simulink model "aaa"  (R2016b)
settings: Solver=ode4  StartTime=0.0  StopTime=inf  FixedStep=0.002  RelTol=1e-3  EnableMultiTasking=on
undefined symbols (not defined in the file or in its folder): bit, mdaadlink6208, sigbuilder_block, Standard
libraries: slrtlib x20, slrtsoftinglib x11, simulink x10
(part 3 of 4)

== system aaa/Subsystem2/zidong/Subsystem ==
  kaigaikaishi : Inport
  guangaikaishi : Inport  Port=2
  kaigaiquxian : Inport  Port=3
  guangaiquxian : Inport  Port=4
  xkgg : Inport  Port=5
  Add1 : Sum
  Constant : Constant  Value=2
  Constant1 : Constant  Value=-0.05
  Display{,1..3} (4 alike) : Display
  Gain : Gain  Gain=0.15
  Gain1 : Gain  Gain=0.15
  Multiport Switch : MultiPortSwitch
  Product : Product
  Sum : Sum  Inputs=|+-
  Sum1 : Sum  Inputs=|+-
  Out1 : Outport
  wires:
  guangaikaishi/1 -> Product/1
  Constant/1 -> Product/2
  kaigaikaishi/1 -> Add1/1
  Product/1 -> Add1/2
  Add1/1 -> Multiport Switch/1
  Multiport Switch/1 -> Display2/1, Out1/1
  Sum/1 -> Gain/1
  Gain/1 -> Multiport Switch/2, Display1/1
  Sum1/1 -> Gain1/1
  Gain1/1 -> Display/1, Multiport Switch/3
  Constant1/1 -> Multiport Switch/4
  xkgg/1 -> Display3/1, Sum1/2, Sum/2
  kaigaiquxian/1 -> Sum/1
  guangaiquxian/1 -> Sum1/1

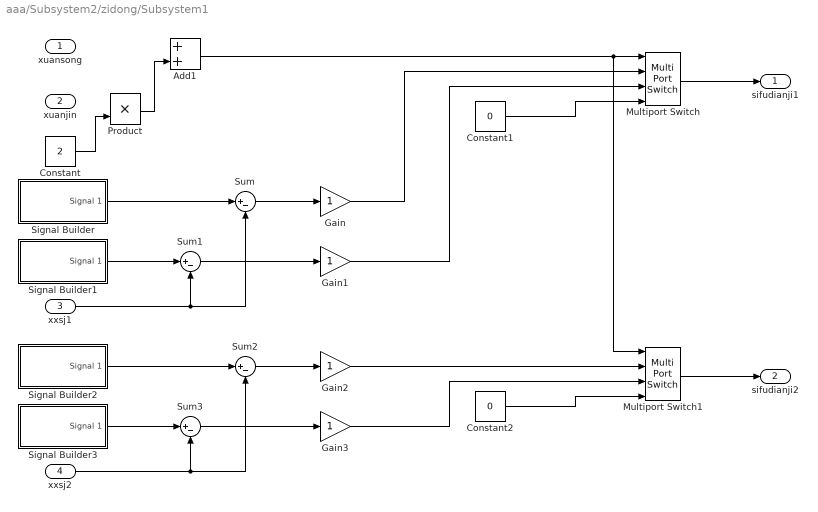
== system aaa/Subsystem2/zidong/Subsystem1 ==
  xuansong : Inport
  xuanjin : Inport  Port=2
  xxsj1 : Inport  Port=3
  xxsj2 : Inport  Port=4
  Add1 : Sum
  Constant : Constant  Value=2
  Constant1 : Constant  Value=0
  Constant2 : Constant  Value=0
  Gain{,1..3} (4 alike) : Gain
  Multiport Switch : MultiPortSwitch
  Multiport Switch1 : MultiPortSwitch
  Product : Product
  Signal Builder : Subsystem  Tag=STV Subsys  LoadFcn=sigbuilder_block('load');  StartFcn=sigbuilder_block('start');  StopFcn=sigbuilder_block('stop');  ClipboardFcn=sigbuilder_block('clipboard');  mask(Sigbuilder block){tuvar=[0:10]}
      mask help: Simulink:masks:SigbuilderBlock_MD
      mask init:
      | if ~strcmp(get_param(bdroot(gcbh),'SimulationStatus'),'stopped') tuvar = sigbuilder_block('maskInit'); end
      settings: CopyFcn=sigbuilder_block('copy');  DeleteFcn=sigbuilder_block('delete');  ModelCloseFcn=sigbuilder_block('modelClose');  PreSaveFcn=sigbuilder_block('preSave');  PauseFcn=sigbuilder_block('pause');  ContinueFcn=sigbuilder_block('continue');  NameChangeFcn=sigbuilder_block('namechange');  OpenFcn=sigbuilder_block('open',[437.6 199.2 550.4 400 ]);  CloseFcn=sigbuilder_block('close');
      mask Display: plot(0, 0, 100, 100,[2, 2, 32, 32, 2], [68, 8, 8, 68, 68],[32, 2], [38, 38], [32, 19, 2],[53, 60, 44], [32, 17, 17, 2],[16, 16, 31, 31]);txt = getActiveGroup(gcbh);text(2, 100, txt,'verticalAlignment', 'top');
  Signal Builder1 : Subsystem  Tag=STV Subsys  LoadFcn=sigbuilder_block('load');  StartFcn=sigbuilder_block('start');  StopFcn=sigbuilder_block('stop');  ClipboardFcn=sigbuilder_block('clipboard');  mask(Sigbuilder block){tuvar=[0:10]}
      mask help: Simulink:masks:SigbuilderBlock_MD
      mask init:
      | if ~strcmp(get_param(bdroot(gcbh),'SimulationStatus'),'stopped') tuvar = sigbuilder_block('maskInit'); end
      settings: CopyFcn=sigbuilder_block('copy');  DeleteFcn=sigbuilder_block('delete');  ModelCloseFcn=sigbuilder_block('modelClose');  PreSaveFcn=sigbuilder_block('preSave');  PauseFcn=sigbuilder_block('pause');  ContinueFcn=sigbuilder_block('continue');  NameChangeFcn=sigbuilder_block('namechange');  OpenFcn=sigbuilder_block('open',[437.6 199.2 550.4 400 ]);  CloseFcn=sigbuilder_block('close');
      mask Display: plot(0, 0, 100, 100,[2, 2, 32, 32, 2], [68, 8, 8, 68, 68],[32, 2], [38, 38], [32, 19, 2],[53, 60, 44], [32, 17, 17, 2],[16, 16, 31, 31]);txt = getActiveGroup(gcbh);text(2, 100, txt,'verticalAlignment', 'top');
  Signal Builder2 : Subsystem  Tag=STV Subsys  LoadFcn=sigbuilder_block('load');  StartFcn=sigbuilder_block('start');  StopFcn=sigbuilder_block('stop');  ClipboardFcn=sigbuilder_block('clipboard');  mask(Sigbuilder block){tuvar=[0:10]}
      mask help: Simulink:masks:SigbuilderBlock_MD
      mask init:
      | if ~strcmp(get_param(bdroot(gcbh),'SimulationStatus'),'stopped') tuvar = sigbuilder_block('maskInit'); end
      settings: CopyFcn=sigbuilder_block('copy');  DeleteFcn=sigbuilder_block('delete');  ModelCloseFcn=sigbuilder_block('modelClose');  PreSaveFcn=sigbuilder_block('preSave');  PauseFcn=sigbuilder_block('pause');  ContinueFcn=sigbuilder_block('continue');  NameChangeFcn=sigbuilder_block('namechange');  OpenFcn=sigbuilder_block('open',[437.6 199.2 550.4 400 ]);  CloseFcn=sigbuilder_block('close');
      mask Display: plot(0, 0, 100, 100,[2, 2, 32, 32, 2], [68, 8, 8, 68, 68],[32, 2], [38, 38], [32, 19, 2],[53, 60, 44], [32, 17, 17, 2],[16, 16, 31, 31]);txt = getActiveGroup(gcbh);text(2, 100, txt,'verticalAlignment', 'top');
  Signal Builder3 : Subsystem  Tag=STV Subsys  LoadFcn=sigbuilder_block('load');  StartFcn=sigbuilder_block('start');  StopFcn=sigbuilder_block('stop');  ClipboardFcn=sigbuilder_block('clipboard');  mask(Sigbuilder block){tuvar=[0:10]}
      mask help: Simulink:masks:SigbuilderBlock_MD
      mask init:
      | if ~strcmp(get_param(bdroot(gcbh),'SimulationStatus'),'stopped') tuvar = sigbuilder_block('maskInit'); end
      settings: CopyFcn=sigbuilder_block('copy');  DeleteFcn=sigbuilder_block('delete');  ModelCloseFcn=sigbuilder_block('modelClose');  PreSaveFcn=sigbuilder_block('preSave');  PauseFcn=sigbuilder_block('pause');  ContinueFcn=sigbuilder_block('continue');  NameChangeFcn=sigbuilder_block('namechange');  OpenFcn=sigbuilder_block('open',[437.6 199.2 550.4 400 ]);  CloseFcn=sigbuilder_block('close');
      mask Display: plot(0, 0, 100, 100,[2, 2, 32, 32, 2], [68, 8, 8, 68, 68],[32, 2], [38, 38], [32, 19, 2],[53, 60, 44], [32, 17, 17, 2],[16, 16, 31, 31]);txt = getActiveGroup(gcbh);text(2, 100, txt,'verticalAlignment', 'top');
  Sum{,1..3} (4 alike) : Sum  Inputs=|+-
  sifudianji1 : Outport
  sifudianji2 : Outport  Port=2
  wires:
  Constant1/1 -> Multiport Switch/4
  Gain1/1 -> Multiport Switch/3
  Sum1/1 -> Gain1/1
  Signal Builder1/1(Signal 1) -> Sum1/1
  Gain/1 -> Multiport Switch/2
  Sum/1 -> Gain/1
  xxsj1/1 -> Sum/2, Sum1/2
  Signal Builder/1(Signal 1) -> Sum/1
  Multiport Switch/1 -> sifudianji1/1
  Add1/1 -> Multiport Switch1/1, Multiport Switch/1
  Product/1 -> Add1/2
  Constant/1 -> Product/2
  Multiport Switch1/1 -> sifudianji2/1
  Signal Builder2/1(Signal 1) -> Sum2/1
  xxsj2/1 -> Sum2/2, Sum3/2
  Sum2/1 -> Gain2/1
  Gain2/1 -> Multiport Switch1/2
  Signal Builder3/1(Signal 1) -> Sum3/1
  Sum3/1 -> Gain3/1
  Gain3/1 -> Multiport Switch1/3
  Constant2/1 -> Multiport Switch1/4

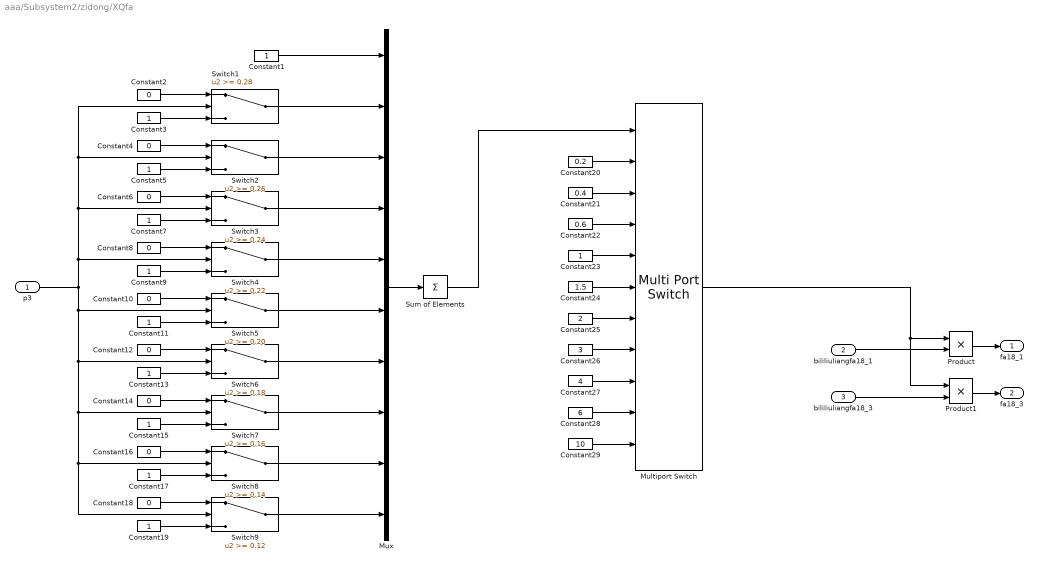
== system aaa/Subsystem2/zidong/XQfa ==
  p3 : Inport
  bililiuliangfa18_1 : Inport  Port=2
  bililiuliangfa18_3 : Inport  Port=3
  Constant{1,3,5,7,9,11,13,15,17,19,23} (11 alike) : Constant
  Constant{2,4,6,8,10,12,14,16,18} (9 alike) : Constant  Value=0
  Constant20 : Constant  Value=0.2
  Constant21 : Constant  Value=0.4
  Constant22 : Constant  Value=0.6
  Constant24 : Constant  Value=1.5
  Constant25 : Constant  Value=2
  Constant26 : Constant  Value=3
  Constant27 : Constant  Value=4
  Constant28 : Constant  Value=6
  Constant29 : Constant  Value=10
  Multiport Switch : MultiPortSwitch  Inputs=10
  Mux : Mux  Inputs=10
  Product : Product  RndMeth=Zero
  Product1 : Product  RndMeth=Zero
  Sum of Elements : Sum  Inputs=+
  Switch1 : Switch  Threshold=0.28
  Switch2 : Switch  Threshold=0.26
  Switch3 : Switch  Threshold=0.24
  Switch4 : Switch  Threshold=0.22
  Switch5 : Switch  Threshold=0.20
  Switch6 : Switch  Threshold=0.18
  Switch7 : Switch  Threshold=0.16
  Switch8 : Switch  Threshold=0.14
  Switch9 : Switch  Threshold=0.12
  fa18_1 : Outport
  fa18_3 : Outport  Port=2
  wires:
  Constant2/1 -> Switch1/1
  Constant3/1 -> Switch1/3
  Constant4/1 -> Switch2/1
  Constant5/1 -> Switch2/3
  Constant6/1 -> Switch3/1
  Constant7/1 -> Switch3/3
  Constant8/1 -> Switch4/1
  Constant9/1 -> Switch4/3
  Constant10/1 -> Switch5/1
  Constant11/1 -> Switch5/3
  Constant12/1 -> Switch6/1
  Constant13/1 -> Switch6/3
  Constant14/1 -> Switch7/1
  Constant15/1 -> Switch7/3
  p3/1 -> Switch1/2, Switch2/2, Switch3/2, Switch4/2, Switch6/2, Switch7/2, Switch8/2, Switch9/2, Switch5/2
  Mux/1 -> Sum of Elements/1
  Sum of Elements/1 -> Multiport Switch/1
  Constant1/1 -> Mux/1
  Switch1/1 -> Mux/2
  Switch2/1 -> Mux/3
  Switch3/1 -> Mux/4
  Switch4/1 -> Mux/5
  Switch5/1 -> Mux/6
  Switch6/1 -> Mux/7
  Switch7/1 -> Mux/8
  Switch8/1 -> Mux/9
  Switch9/1 -> Mux/10
  Constant16/1 -> Switch8/1
  Constant17/1 -> Switch8/3
  Constant18/1 -> Switch9/1
  Constant19/1 -> Switch9/3
  Multiport Switch/1 -> Product/1, Product1/1
  Constant20/1 -> Multiport Switch/2
  Constant21/1 -> Multiport Switch/3
  Constant22/1 -> Multiport Switch/4
  Constant23/1 -> Multiport Switch/5
  Constant24/1 -> Multiport Switch/6
  Constant25/1 -> Multiport Switch/7
  Constant26/1 -> Multiport Switch/8
  Constant27/1 -> Multiport Switch/9
  Constant28/1 -> Multiport Switch/10
  Constant29/1 -> Multiport Switch/11
  bililiuliangfa18_1/1 -> Product/2
  bililiuliangfa18_3/1 -> Product1/2
  Product/1 -> fa18_1/1
  Product1/1 -> fa18_3/1

== system aaa/Subsystem2/shoudong/Subsystem2/Signal Builder ==
  Demux : Demux  Tag=STV Demux  Outputs=1
  FromWs : FromWorkspace  Tag=STV FromWs  VariableName=tuvar  SampleTime=0
      SigBuilderData=|
      | common.afterFinalStr = 'Extrapolate'
      | common.sampleTime = 0
      | dataSet.timeRange = [0 10]
      | dataSet.name = 'Group 1'
      | sbobj.Groups.Name = 'Group 1'
      | sbobj.Groups.Signals.Name = 'Signal 1'
      | sbobj.Groups.Signals.XData = [0 4 4 6 6 10]
      | sbobj.Groups.Signals.YData = [0 0 1 1 0 0]
  Signal 1 : Outport  Tag=STV Outport
  wires:
  FromWs/1 -> Demux/1
  Demux/1 -> Signal 1/1

== system aaa/Subsystem2/shoudong/Subsystem2/Signal Builder1 ==
  Demux : Demux  Tag=STV Demux  Outputs=1
  FromWs : FromWorkspace  Tag=STV FromWs  VariableName=tuvar  SampleTime=0
      SigBuilderData=|
      | common.afterFinalStr = 'Extrapolate'
      | common.sampleTime = 0
      | dataSet.timeRange = [0 10]
      | dataSet.name = 'Group 1'
      | sbobj.Groups.Name = 'Group 1'
      | sbobj.Groups.Signals.Name = 'Signal 1'
      | sbobj.Groups.Signals.XData = [0 4 4 6 6 10]
      | sbobj.Groups.Signals.YData = [0 0 1 1 0 0]
  Signal 1 : Outport  Tag=STV Outport
  wires:
  Demux/1 -> Signal 1/1
  FromWs/1 -> Demux/1

== system aaa/Subsystem2/shoudong/Subsystem2/Signal Builder2 ==
  Demux : Demux  Tag=STV Demux  Outputs=1
  FromWs : FromWorkspace  Tag=STV FromWs  VariableName=tuvar  SampleTime=0
      SigBuilderData=|
      | common.afterFinalStr = 'Extrapolate'
      | common.sampleTime = 0
      | dataSet.timeRange = [0 10]
      | dataSet.name = 'Group 1'
      | sbobj.Groups.Name = 'Group 1'
      | sbobj.Groups.Signals.Name = 'Signal 1'
      | sbobj.Groups.Signals.XData = [0 4 4 6 6 10]
      | sbobj.Groups.Signals.YData = [0 0 1 1 0 0]
  Signal 1 : Outport  Tag=STV Outport
  wires:
  Demux/1 -> Signal 1/1
  FromWs/1 -> Demux/1

== system aaa/Subsystem2/shoudong/Subsystem2/Signal Builder3 ==
  Demux : Demux  Tag=STV Demux  Outputs=1
  FromWs : FromWorkspace  Tag=STV FromWs  VariableName=tuvar  SampleTime=0
      SigBuilderData=|
      | common.afterFinalStr = 'Extrapolate'
      | common.sampleTime = 0
      | dataSet.timeRange = [0 10]
      | dataSet.name = 'Group 1'
      | sbobj.Groups.Name = 'Group 1'
      | sbobj.Groups.Signals.Name = 'Signal 1'
      | sbobj.Groups.Signals.XData = [0 4 4 6 6 10]
      | sbobj.Groups.Signals.YData = [0 0 1 1 0 0]
  Signal 1 : Outport  Tag=STV Outport
  wires:
  FromWs/1 -> Demux/1
  Demux/1 -> Signal 1/1

== system aaa/Subsystem2/zidong/Subsystem1/Signal Builder ==
  Demux : Demux  Tag=STV Demux  Outputs=1
  FromWs : FromWorkspace  Tag=STV FromWs  VariableName=tuvar  SampleTime=0
      SigBuilderData=|
      | common.afterFinalStr = 'Extrapolate'
      | common.sampleTime = 0
      | dataSet.timeRange = [0 10]
      | dataSet.name = 'Group 1'
      | sbobj.Groups.Name = 'Group 1'
      | sbobj.Groups.Signals.Name = 'Signal 1'
      | sbobj.Groups.Signals.XData = [0 4 4 6 6 10]
      | sbobj.Groups.Signals.YData = [0 0 1 1 0 0]
  Signal 1 : Outport  Tag=STV Outport
  wires:
  FromWs/1 -> Demux/1
  Demux/1 -> Signal 1/1

== system aaa/Subsystem2/zidong/Subsystem1/Signal Builder1 ==
  Demux : Demux  Tag=STV Demux  Outputs=1
  FromWs : FromWorkspace  Tag=STV FromWs  VariableName=tuvar  SampleTime=0
      SigBuilderData=|
      | common.afterFinalStr = 'Extrapolate'
      | common.sampleTime = 0
      | dataSet.timeRange = [0 10]
      | dataSet.name = 'Group 1'
      | sbobj.Groups.Name = 'Group 1'
      | sbobj.Groups.Signals.Name = 'Signal 1'
      | sbobj.Groups.Signals.XData = [0 4 4 6 6 10]
      | sbobj.Groups.Signals.YData = [0 0 1 1 0 0]
  Signal 1 : Outport  Tag=STV Outport
  wires:
  Demux/1 -> Signal 1/1
  FromWs/1 -> Demux/1

== system aaa/Subsystem2/zidong/Subsystem1/Signal Builder2 ==
  Demux : Demux  Tag=STV Demux  Outputs=1
  FromWs : FromWorkspace  Tag=STV FromWs  VariableName=tuvar  SampleTime=0
      SigBuilderData=|
      | common.afterFinalStr = 'Extrapolate'
      | common.sampleTime = 0
      | dataSet.timeRange = [0 10]
      | dataSet.name = 'Group 1'
      | sbobj.Groups.Name = 'Group 1'
      | sbobj.Groups.Signals.Name = 'Signal 1'
      | sbobj.Groups.Signals.XData = [0 4 4 6 6 10]
      | sbobj.Groups.Signals.YData = [0 0 1 1 0 0]
  Signal 1 : Outport  Tag=STV Outport
  wires:
  Demux/1 -> Signal 1/1
  FromWs/1 -> Demux/1

== system aaa/Subsystem2/zidong/Subsystem1/Signal Builder3 ==
  Demux : Demux  Tag=STV Demux  Outputs=1
  FromWs : FromWorkspace  Tag=STV FromWs  VariableName=tuvar  SampleTime=0
      SigBuilderData=|
      | common.afterFinalStr = 'Extrapolate'
      | common.sampleTime = 0
      | dataSet.timeRange = [0 10]
      | dataSet.name = 'Group 1'
      | sbobj.Groups.Name = 'Group 1'
      | sbobj.Groups.Signals.Name = 'Signal 1'
      | sbobj.Groups.Signals.XData = [0 4 4 6 6 10]
      | sbobj.Groups.Signals.YData = [0 0 1 1 0 0]
  Signal 1 : Outport  Tag=STV Outport
  wires:
  FromWs/1 -> Demux/1
  Demux/1 -> Signal 1/1

== stateflow chart aaa/Subsystem2/zidong/Chart ==
  state zidong
    state SXQxieya
      state off1
        entry:
        diancifa11_1=0;
        bililiuliangfa18_3=0;
        bililiuliangfa18_4=0;
      state on1
        entry:
        diancifa11_5=1;
      state xieya1
        entry:
        bililiuliangfa18_1=1;
        bililiuliangfa18_2=1;
        p0_2=p0sheding;
      state xieya1_2
        entry:
        bililiuliangfa18_1=1;
        bililiuliangfa18_2=0;
      state xieya1_1
        entry:
        bililiuliangfa18_1=1;
        bililiuliangfa18_2=1;
      state xieya1_3
        entry:
        bililiuliangfa18_1=0;
        bililiuliangfa18_2=1;
      state xieya2
        entry:
        bililiuliangfa18_1=1;
        bililiuliangfa18_2=1;
        p0_2=p0_2-0.03;
      state xieya7_2
        entry:
        bililiuliangfa18_1=1;
        bililiuliangfa18_2=0;
      state xieya7_1
        entry:
        bililiuliangfa18_1=1;
        bililiuliangfa18_2=1;
      state xieya7_3
        entry:
        bililiuliangfa18_1=0;
        bililiuliangfa18_2=1;
      state off2
        entry:
        diancifa11_5=0;
        bililiuliangfa18_1=0;
        bililiuliangfa18_2=0;
        SXQxieyawancheng=1;
      state xieya8
        entry:
        bililiuliangfa18_1=1;
        bililiuliangfa18_2=1;
      (default) -> zidong.SXQxieya.off1
      zidong.SXQxieya.off1 -> zidong.SXQxieya.on1
      zidong.SXQxieya.on1 -> xieya1 : after(20,tick)
      xieya1 -> (junction 1107)
      (junction 1107) -> xieya1_2 [order 2] : [p2<=p0_2&&p3>p0_2]
      (junction 1107) -> xieya1_1 [order 1] : [p2>p0_2&&p3>p0_2]
      xieya1_2 -> (junction 1107)
      xieya1_3 -> (junction 1107)
      xieya1_1 -> (junction 1107)
      (junction 1107) -> xieya1_3 [order 3] : [p2>p0_2&&p3<=p0_2]
      (junction 1107) -> xieya2 [order 4] : [p2<=p0_2&&p3<=p0_2]
      (junction 1108) -> (junction 1107) [order 2] : [p0_2>p0_0]
      xieya2 -> (junction 1108)
      (junction 1108) -> (junction 1109) [order 1] : [p0_2<=p0_0]
      (junction 1109) -> xieya7_2 [order 2] : [p2<=p0_0&&p3>p0_0]
      xieya7_2 -> (junction 1109)
      (junction 1109) -> xieya7_1 [order 1] : [p2>p0_0&&p3>p0_0]
      xieya7_3 -> (junction 1109)
      (junction 1109) -> xieya7_3 [order 3] : [p2>p0_0&&p3<=p0_0]
      xieya7_1 -> (junction 1109)
      (junction 1109) -> xieya8 [order 4] : [p2<=p0_0&&p3<=p0_0]
      (junction 1110) -> (junction 1109) [order 2] : [p2>p0_0||p3>p0_0]
      (junction 1110) -> zidong.SXQxieya.off2 [order 1] : [p2<=p0_0&&p3<=p0_0]
      xieya8 -> (junction 1110) : after(1000,tick)
    state kaiguangai
      state start
        entry:
        xuansong=0;
        xuanjin=0;
        suoding=0;
        jiesuo=0;
        kaigaikaishi=0;
        guangaikaishi=0;
        diancifa20=0;
      state on5
        entry:
        jiesuo=1;
        xuansong=1;
      state off5
        entry:
        jiesuo=0;
        xuansong=0;
      state on1
        entry:diancifa20=1;
      state on6
        entry:
        guangaikaishi=1;
      state on2
        entry:
        xuansong=1;
        jiesuo=1;
      state on7
        entry:
        guangaikaishi=0;
        diancifa20=1;
      state off1
        entry:
        xuansong=0;
        jiesuo=0;
      state on8
        entry:
        xuanjin=1;
      state off2
        entry:
        diancifa20=0;
        SQshiyabuchangwancheng=1;
      state off6
        entry:
        xuanjin=0;
      state on3
        entry:
        kaigaikaishi=1;
      state on4
        entry:
        kaigaikaishi=0;
        suoding=1;
      state off7
        entry:
        diancifa20=0;
        SQxuanjinjianyawancheng=1;
        guangaiwancheng=1;
      state off3
        entry:
        suoding=0;
      state off4
        entry:
        kaigaiwancheng=1;
      (default) -> zidong.kaiguangai.start
      zidong.kaiguangai.off4 -> on5 : after(2500,tick)
      on5 -> off5 : [jiesuodaowei1==1&&jiesuodaowei2==1&&xuansongdaowei1==1&&xuansongdaowei2==1]
      zidong.kaiguangai.start -> zidong.kaiguangai.on1
      off5 -> on6 : after(500,tick)
      zidong.kaiguangai.on1 -> zidong.kaiguangai.on2 : [liuliangji==1&&p1>=p2-0.01&&p1<=p2+0.01]
      on6 -> on7 : [guangaijieshu==1]
      zidong.kaiguangai.on2 -> zidong.kaiguangai.off1 : [xuansongdaowei1==1&&xuansongdaowei2==1&&jiesuodaowei1==1&&jiesuodaowei2==1]
      on7 -> on8
      zidong.kaiguangai.off1 -> zidong.kaiguangai.off2 : after(20,tick)
      on8 -> zidong.kaiguangai.off6 : [xuanjindaowei1==1&&xuanjindaowei2==1]
      zidong.kaiguangai.off2 -> zidong.kaiguangai.on3 : after(500,tick)
      zidong.kaiguangai.off6 -> off7 : after(20,tick)
      zidong.kaiguangai.on3 -> on4 : [kaigaijieshu==1]
      on4 -> zidong.kaiguangai.off3 : [suodingdaowei1==1&&suodingdaowei2==1]
      zidong.kaiguangai.off3 -> zidong.kaiguangai.off4 : after(20,tick)
    state SCjiaya
      state off1
        entry:diancifa11_1=0;
        diancifa11_2=0;
        diancifa16_1=0;
      state on1
        entry:diancifa11_1=1;
        diancifa11_2=1;
        diancifa16_1=0;
      state off2
        entry:
        diancifa11_1=0;
        diancifa11_2=0;
        diancifa16_1=0;
      state on3
        entry:diancifa11_1=1;
        diancifa11_2=1;
        diancifa16_1=0;
      state on2
        entry:diancifa16_1=1;
      state off3
        entry:
        diancifa11_1=0;
        diancifa11_2=0;
        diancifa16_1=0;
      state off4
        entry:
        SCjiayawancheng=1;
      (default) -> zidong.SCjiaya.off1
      zidong.SCjiaya.off1 -> zidong.SCjiaya.on1
      zidong.SCjiaya.on1 -> zidong.SCjiaya.off2 : [p1>=p1sheding]
      zidong.SCjiaya.off2 -> (junction 45) : after(1000,tick)
      zidong.SCjiaya.on2 -> (junction 45)
      zidong.SCjiaya.on3 -> (junction 45)
      (junction 45) -> zidong.SCjiaya.on2 [order 2] : [p1>p1sheding+0.005]
      (junction 45) -> zidong.SCjiaya.on3 [order 1] : [p1<p1sheding]
      (junction 45) -> zidong.SCjiaya.off3 [order 3] : [p1>=p1sheding&&p1<=p1sheding+0.005]
      zidong.SCjiaya.off3 -> zidong.SCjiaya.off4
    state SCzhushui
      state off4
        entry:diancifa16_1=0;
        diancifa3=0;
      state on2
        entry:diancifa16_1=1;
      state on3
        entry:diancifa3=1;
      state off1
        entry:diancifa3=0;
      state off2
        entry:diancifa16_1=0;
      state off3
        entry:
        SCzhushuiwancheng=1;
      (default) -> zidong.SCzhushui.off4
      zidong.SCzhushui.off4 -> zidong.SCzhushui.on2
      zidong.SCzhushui.on2 -> zidong.SCzhushui.on3 : after(20,tick)
      zidong.SCzhushui.on3 -> zidong.SCzhushui.off1 : [fuqiuyeweikongzhiqi==1]
      zidong.SCzhushui.off1 -> zidong.SCzhushui.off2
      zidong.SCzhushui.off2 -> zidong.SCzhushui.off3
    state SXQjunya
      state jiaya1_1
        entry:
        bililiuliangfa18_3=1;
        bililiuliangfa18_4=1;
      state jiaya7_1
        entry:
        bililiuliangfa18_3=1;
        bililiuliangfa18_4=1;
      state jiaya7_3
        entry:
        bililiuliangfa18_3=0;
        bililiuliangfa18_4=1;
      state jiaya2
        entry:
        bililiuliangfa18_3=1;
        bililiuliangfa18_4=1;
        p0_1=p0_1+0.03;
      state off1
        entry:
        diancifa11_1=0;
        diancifa11_5=0;
        diancifa20=0;
        bililiuliangfa18_1=0;
        bililiuliangfa18_2=0;
        bililiuliangfa18_3=0;
        bililiuliangfa18_4=0;
      state jiaya1
        entry:
        bililiuliangfa18_3=1;
        bililiuliangfa18_4=1;
        p0_1=p0_0;
      state on1
        entry:
        diancifa11_1=1;
        diancifa11_5=1;
      state jiaya7_2
        entry:
        bililiuliangfa18_3=1;
        bililiuliangfa18_4=0;
      state jiaya1_2
        entry:
        bililiuliangfa18_3=1;
        bililiuliangfa18_4=0;
      state jiaya1_3
        entry:
        bililiuliangfa18_3=0;
        bililiuliangfa18_4=1;
      state off4
        entry:
        bililiuliangfa18_3=0;
        bililiuliangfa18_4=0;
      state off3
        entry:
        bililiuliangfa18_1=0;
        bililiuliangfa18_2=0;
      state off2
        entry:
        bililiuliangfa18_1=0;
        bililiuliangfa18_2=0;
        bililiuliangfa18_3=0;
        bililiuliangfa18_4=0;
      state jiance1_34
        entry:
        bililiuliangfa18_1=1;
        bililiuliangfa18_2=0;
      state jiance1_32
        entry:
        bililiuliangfa18_1=1;
        bililiuliangfa18_2=1;
      state jiance1_36
        entry:
        bililiuliangfa18_1=0;
        bililiuliangfa18_2=1;
      state off6
        entry:
        diancifa11_1=0;
        diancifa11_5=0;
        SXQjunyawancheng=1;
      jiaya1_1 -> (junction 1195)
      jiaya7_3 -> (junction 1197)
      (junction 1195) -> jiaya2 [order 4] : [p2>=p0_1&&p3>=p0_1]
      (junction 1197) -> jiaya7_1 [order 1] : [p2<p0sheding&&p3<p0sheding]
      (default) -> zidong.SXQjunya.off1
      (junction 1195) -> jiaya1_1 [order 1] : [p2<p0_1&&p3<p0_1]
      jiaya7_1 -> (junction 1197)
      (junction 1197) -> jiaya7_3 [order 3] : [p2<p0sheding&&p3>=p0sheding]
      jiaya2 -> (junction 1196)
      (junction 1197) -> jiaya7_2 [order 2] : [p2>=p0sheding&&p3<p0sheding]
      jiaya1 -> (junction 1195)
      (junction 1196) -> (junction 1195) [order 2] : [p0_1<p0sheding]
      (junction 1196) -> (junction 1197) [order 1] : [p0_1>=p0sheding]
      (junction 1195) -> jiaya1_3 [order 3] : [p2<p0_1&&p3>=p0_1]
      jiaya7_2 -> (junction 1197)
      zidong.SXQjunya.on1 -> jiaya1 : after(500,tick)
      zidong.SXQjunya.off1 -> zidong.SXQjunya.on1
      jiaya1_3 -> (junction 1195)
      (junction 1195) -> jiaya1_2 [order 2] : [p2>=p0_1&&p3<p0_1]
      zidong.SXQjunya.off4 -> (junction 1197) [order 2] : [p2<p0sheding||p3<p0sheding]
      zidong.SXQjunya.off3 -> (junction 1197) [order 2] : [p2<=(p0sheding+0.005)&&p3<=(p0sheding+0.005)]
      jiaya1_2 -> (junction 1195)
      (junction 1197) -> zidong.SXQjunya.off4 [order 4] : after(250,tick)[p2>=p0sheding&&p3>=p0sheding]
      (junction 1198) -> zidong.SXQjunya.off3 [order 5] : after(250,tick)[p2<=(p0sheding+0.005)&&p3<=(p0sheding+0.005)]
      zidong.SXQjunya.off4 -> (junction 1198) [order 1]
      zidong.SXQjunya.off3 -> (junction 1198) [order 1] : [p2>(p0sheding+0.005)||p3>(p0sheding+0.005)]
      (junction 1198) -> jiance1_34 [order 1] : [p2<=(p0sheding+0.005)&&p3>(p0sheding+0.005)]
      (junction 1198) -> zidong.SXQjunya.off2 [order 2] : [p2>=p0sheding&&p3>=p0sheding&&p2<=(p0sheding+0.005)&&p3<=(p0sheding+0.005)]
      jiance1_34 -> (junction 1198)
      (junction 1199) -> (junction 1198) [order 1] : [p2<p0sheding||p2>(p0sheding+0.005)||p3<p0sheding||p3>(p0sheding+0.005)]
      jiance1_32 -> (junction 1198)
      (junction 1198) -> jiance1_36 [order 3] : [p2>(p0sheding+0.005)&&p3<=(p0sheding+0.005)]
      jiance1_36 -> (junction 1198)
      (junction 1198) -> jiance1_32 [order 4] : [p2>(p0sheding+0.005)&&p3>(p0sheding+0.005)]
      zidong.SXQjunya.off2 -> (junction 1199) : after(1000,tick)
      (junction 1199) -> zidong.SXQjunya.off6 [order 2] : [p2>=p0sheding&&p2<=(p0sheding+0.005)&&p3>=p0sheding&&p3<=(p0sheding+0.005)]
    (default) -> SCzhushui
    zidong.SCzhushui.off3 -> SCjiaya : after(1000,tick)
    off7 -> SXQxieya : after(1000,tick)
    zidong.SCjiaya.off4 -> SXQjunya : after(1000,tick)
    zidong.SXQjunya.off6 -> kaiguangai : after(1000,tick)
  state start
    en:
    diancifa11_1=0;
    diancifa11_2=0;
    diancifa11_5=0;
    diancifa20=0;
    diancifa16_1=0;
    diancifa3=0;
    diancifa21=0;
    bililiuliangfa18_1=0;
    bililiuliangfa18_2=0;
    bililiuliangfa18_3=0;
    bililiuliangfa18_4=0;
    xuansong=0;
    xuanjin=0;
    suoding=0;
    jiesuo=0;
    kaigaikaishi=0;
    guangaikaishi=0;
  state off111
    en:
    diancifa11_1=0;
    diancifa11_2=0;
    diancifa11_5=0;
    diancifa20=0
    diancifa16_1=0;
    diancifa3=0;
    diancifa21=0;
    bililiuliangfa18_1=0;
    bililiuliangfa18_2=0;
    bililiuliangfa18_3=0;
    bililiuliangfa18_4=0;
    xuansong=0;
    xuanjin=0;
    suoding=0;
    jiesuo=0;
    SCzhushuiwancheng=0;
    SCjiayawancheng=0;
    SXQjunyawancheng=0;
    SQshiyabuchangwancheng=0;
    kaigaikaishi=0;
    kaigaiwancheng=0;
    SQxuanjinjianyawancheng=0;
    guangaikaishi=0;
    guangaiwancheng=0;
    SXQxieyawancheng=0;
  (default) -> start
  start -> zidong : [start==1]
  off111 -> start : [start==0&&jiting==0]
  zidong -> off111 : [jiting==1||start==0]
  data: start input double; diancifa11_1 output double; diancifa11_2 output double; diancifa11_5 output double; SCzhushui input double; fuqiuyeweikongzhiqi input double; diancifa20 output double; diancifa16_1 output double; diancifa3 output double; SCjiaya input double; SXQjunya input double; diancifa21 output double; suoding output double; jiesuo output double; xuansong output double; xuanjin output double; bililiuliangfa18_1 output double; bililiuliangfa18_2 output double; bililiuliangfa18_3 output double; bililiuliangfa18_4 output double; SXQxieya input double; p1 input double; p1sheding input double; liuliangji input double; p2 input double; p3 input double; p0_0 input double; p0sheding input double; kaigaikaishi output double; guangaikaishi output double; SCzhushuiwancheng output double; SCjiayawancheng output double; SXQjunyawancheng output double; SXQxieyawancheng output double; SQshiyabuchangwancheng output double; SQxuanjinjianyawancheng output double; kaigaiwancheng output double; guangaiwancheng output double; xuansongdaowei1 input double; xuansongdaowei2 input double; xuanjindaowei1 input double; xuanjindaowei2 input double; suodingdaowei1 input double; suodingdaowei2 input double; jiesuodaowei1 input double; jiesuodaowei2 input double; kaigaijieshu input double; guangaijieshu input double; p0_1 local double; p0_2 local double; jiting input double; zidongkaigai input double; zidongguangai input double

== stateflow chart aaa/jinjichuli/jinjichuli ==
  state MANUAL
    state fa4_4 [parallel]
      settings: executionOrder=1
      state A
        entry:diancifa20=0;
      state on
        entry:diancifa20=1;
      (default) -> MANUAL.fa4_4.A
      MANUAL.fa4_4.on -> MANUAL.fa4_4.A : [fa20==0]
      MANUAL.fa4_4.A -> MANUAL.fa4_4.on : [fa20==1]
    state fa4_2 [parallel]
      settings: executionOrder=2
      state A
        entry:diancifa11_2=0;
      state on
        entry:diancifa11_2=1;
      (default) -> MANUAL.fa4_2.A
      MANUAL.fa4_2.on -> MANUAL.fa4_2.A : [fa11_2==0]
      MANUAL.fa4_2.A -> MANUAL.fa4_2.on : [fa11_2==1]
    state fa4_3 [parallel]
      settings: executionOrder=3
      state A
        entry:diancifa11_5=0;
      state on
        entry:diancifa11_5=1;
      (default) -> MANUAL.fa4_3.A
      MANUAL.fa4_3.on -> MANUAL.fa4_3.A : [fa11_5==0]
      MANUAL.fa4_3.A -> MANUAL.fa4_3.on : [fa11_5==1]
    state fa4_1 [parallel]
      settings: executionOrder=4
      state A
        entry:diancifa11_1=0;
      state on
        entry:diancifa11_1=1;
      (default) -> MANUAL.fa4_1.A
      MANUAL.fa4_1.on -> MANUAL.fa4_1.A : [fa11_1==0]
      MANUAL.fa4_1.A -> MANUAL.fa4_1.on : [fa11_1==1]
    state fa4_5 [parallel]
      settings: executionOrder=5
      state A
        entry:diancifa16_1=0;
      state on
        entry:diancifa16_1=1;
      (default) -> MANUAL.fa4_5.A
      MANUAL.fa4_5.on -> MANUAL.fa4_5.A : [fa16_1==0]
      MANUAL.fa4_5.A -> MANUAL.fa4_5.on : [fa16_1==1]
    state fa4_6 [parallel]
      settings: executionOrder=6
      state A
        entry:diancifa3=0;
      state on
        entry:diancifa3=1;
      (default) -> MANUAL.fa4_6.A
      MANUAL.fa4_6.on -> MANUAL.fa4_6.A : [fa3==0]
      MANUAL.fa4_6.A -> MANUAL.fa4_6.on : [fa3==1]
    state fa4_8 [parallel]
      settings: executionOrder=7
      state A
        entry:xuansong=0;
      state on
        entry:xuansong=1;
      (default) -> MANUAL.fa4_8.A
      MANUAL.fa4_8.on -> MANUAL.fa4_8.A : [xuansongmingling==0]
      MANUAL.fa4_8.A -> MANUAL.fa4_8.on : [xuansongmingling==1]
    state fa4_7 [parallel]
      settings: executionOrder=8
      state A
        entry:diancifa21=0;
      state on
        entry:diancifa21=1;
      (default) -> MANUAL.fa4_7.A
      MANUAL.fa4_7.on -> MANUAL.fa4_7.A : [fa21==0]
      MANUAL.fa4_7.A -> MANUAL.fa4_7.on : [fa21==1]
    state fa4_9 [parallel]
      settings: executionOrder=9
      state A
        entry:xuanjin=0;
      state on
        entry:xuanjin=1;
      (default) -> MANUAL.fa4_9.A
      MANUAL.fa4_9.on -> MANUAL.fa4_9.A : [xuanjinmingling==0]
      MANUAL.fa4_9.A -> MANUAL.fa4_9.on : [xuanjinmingling==1]
    state fa4_10 [parallel]
      settings: executionOrder=10
      state A
        entry:suoding=0;
      state on
        entry:suoding=1;
      (default) -> MANUAL.fa4_10.A
      MANUAL.fa4_10.on -> MANUAL.fa4_10.A : [suodingmingling==0]
      MANUAL.fa4_10.A -> MANUAL.fa4_10.on : [suodingmingling==1]
    state fa4_12 [parallel]
      settings: executionOrder=11
      state A
        entry:bililiuliangfa18_1=0;
      state on
        entry:bililiuliangfa18_1=fa18_1;
      (default) -> MANUAL.fa4_12.A
      MANUAL.fa4_12.on -> MANUAL.fa4_12.A [order 2] : [fa18_1==0]
      MANUAL.fa4_12.A -> MANUAL.fa4_12.on : [fa18_1!=0]
      MANUAL.fa4_12.on -> MANUAL.fa4_12.on [order 1] : [fa18_1!=0]
    state fa4_11 [parallel]
      settings: executionOrder=12
      state A
        entry:jiesuo=0;
      state on
        entry:jiesuo=1;
      (default) -> MANUAL.fa4_11.A
      MANUAL.fa4_11.on -> MANUAL.fa4_11.A : [jiesuomingling==0]
      MANUAL.fa4_11.A -> MANUAL.fa4_11.on : [jiesuomingling==1]
    state fa4_13 [parallel]
      settings: executionOrder=13
      state A
        entry:bililiuliangfa18_2=0;
      state on
        entry:bililiuliangfa18_2=fa18_2;
      (default) -> MANUAL.fa4_13.A
      MANUAL.fa4_13.on -> MANUAL.fa4_13.A [order 2] : [fa18_2==0]
      MANUAL.fa4_13.A -> MANUAL.fa4_13.on : [fa18_2!=0]
      MANUAL.fa4_13.on -> MANUAL.fa4_13.on [order 1] : [fa18_2!=0]
    state kiagai [parallel]
      settings: executionOrder=14
      state A
        entry:bililiuliangfa18_3=0;
      state on
        entry:bililiuliangfa18_3=fa18_3;
      (default) -> MANUAL.kiagai.A
      MANUAL.kiagai.on -> MANUAL.kiagai.A [order 2] : [fa18_3==0]
      MANUAL.kiagai.A -> MANUAL.kiagai.on : [fa18_3!=0]
      MANUAL.kiagai.on -> MANUAL.kiagai.on [order 1] : [fa18_3!=0]
    state yajin [parallel]
      settings: executionOrder=15
      state A
        entry:bililiuliangfa18_4=0;
      state on
        entry:bililiuliangfa18_4=fa18_4;
      (default) -> MANUAL.yajin.A
      MANUAL.yajin.on -> MANUAL.yajin.A [order 2] : [fa18_4==0]
      MANUAL.yajin.A -> MANUAL.yajin.on : [fa18_4!=0]
      MANUAL.yajin.on -> MANUAL.yajin.on [order 1] : [fa18_4!=0]
    state kaigai [parallel]
      settings: executionOrder=16
      state A
        entry:kaiguangaifa=0;
      state on
        entry:kaiguangaifa=fa_kgg;
      (default) -> MANUAL.kaigai.A
      MANUAL.kaigai.on -> MANUAL.kaigai.A [order 2] : [fa_kgg==0]
      MANUAL.kaigai.A -> MANUAL.kaigai.on : [fa_kgg!=0]
      MANUAL.kaigai.on -> MANUAL.kaigai.on [order 1] : [fa_kgg!=0]
  state off1
  state on1
    entry:
    diancifa11_1=0;
    diancifa11_2=0;
    diancifa11_5=0;
    diancifa20=0;
    diancifa16_1=0;
    diancifa3=0;
    diancifa21=0;
    xuansong=0;
    xuanjin=0;
    suoding=0;
    jiesuo=0;
    bililiuliangfa18_1=0;
    bililiuliangfa18_2=0;
    bililiuliangfa18_3=0;
    bililiuliangfa18_4=0;
    kaiguangaifa=0;
  state end
    en:
    diancifa11_1=0;
    diancifa11_2=0;
    diancifa11_5=0;
    diancifa20=0;
    diancifa16_1=0;
    diancifa3=0;
    diancifa21=0;
    xuansong=0;
    xuanjin=0;
    suoding=0;
    jiesuo=0;
    bililiuliangfa18_1=0;
    bililiuliangfa18_2=0;
    bililiuliangfa18_3=0;
    bililiuliangfa18_4=0;
    kaiguangaifa=0;
  (default) -> off1
  off1 -> on1 : [tiaoshi==1]
  on1 -> MANUAL : after(500,tick)
  MANUAL -> end : [jiting==1]
  data: tiaoshi input double; diancifa11_1 output double; diancifa11_2 output double; diancifa11_5 output double; diancifa20 output double; diancifa16_1 output double; diancifa3 output double; diancifa21 output double; suoding output double; jiesuo output double; xuansong output double; xuanjin output double; bililiuliangfa18_1 output double; bililiuliangfa18_2 output double; fa11_1 input; fa11_2 input; fa11_5 input; fa20 input; fa16_1 input; fa3 input; fa21 input; suodingmingling input; jiesuomingling input; xuansongmingling input; xuanjinmingling input; fa18_1 input; fa18_2 input; bililiuliangfa18_3 output double; bililiuliangfa18_4 output double; kaiguangaifa output double; fa18_3 input; fa18_4 input; fa_kgg input; jiting input double
